simulink model "FIR_filter"  (R2020b)
settings: Solver=FixedStepDiscrete  StartTime=0.0  StopTime=10.0  FixedStep=1  RelTol=1e-3
settings Model: Creator=Diwakar Reddy  LastModifiedBy=Diwakar Reddy
settings DataIOCC: SaveOutput=off  SaveTime=off

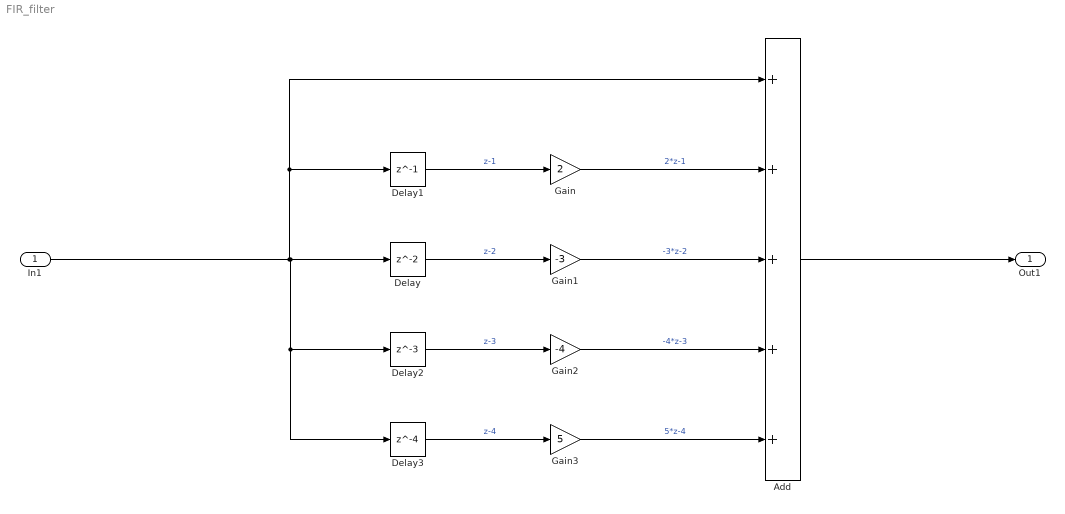
== system FIR_filter ==
  In1 : Inport  OutDataTypeStr=double  PortDimensions=[1 1]  SampleTime=[1,0]
  Add : Sum  Inputs=+++++
  Delay : Delay
  Delay1 : Delay  DelayLength=1
  Delay2 : Delay  DelayLength=3
  Delay3 : Delay  DelayLength=4
  Gain : Gain  Gain=2
  Gain1 : Gain  Gain=-3
  Gain2 : Gain  Gain=-4
  Gain3 : Gain  Gain=5
  Out1 : Outport  OutDataTypeStr=double  PortDimensions=[1 1]  SampleTime=[1,0]
  wires:
  Gain3/1 -> Add/5  "5*z-4"
  Delay2/1 -> Gain2/1  "z-3"
  Gain1/1 -> Add/3  "-3*z-2"
  In1/1 -> Delay/1, Delay2/1, Delay3/1, Delay1/1, Add/1
  Gain/1 -> Add/2  "2*z-1"
  Delay3/1 -> Gain3/1  "z-4"
  Delay/1 -> Gain1/1  "z-2"
  Delay1/1 -> Gain/1  "z-1"
  Gain2/1 -> Add/4  "-4*z-3"
  Add/1 -> Out1/1
